simulink model "InstCamberStiffness"  (R2024b)
settings: Solver=VariableStepAuto  StartTime=0.0  StopTime=30  RelTol=1e-3
libraries: simulink x1
settings Model: Creator=owen  LastModifiedBy=owen

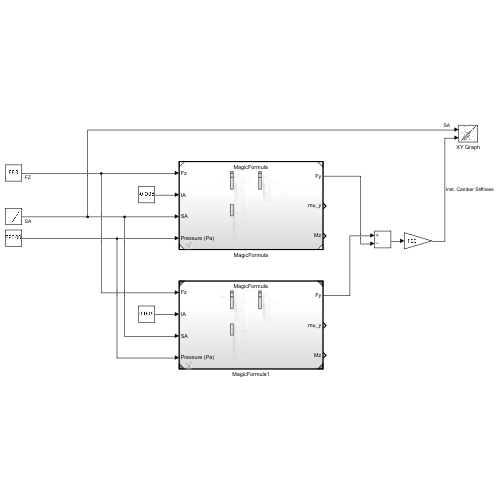
[thumbnail: Simulink's stored preview of the top-level diagram]
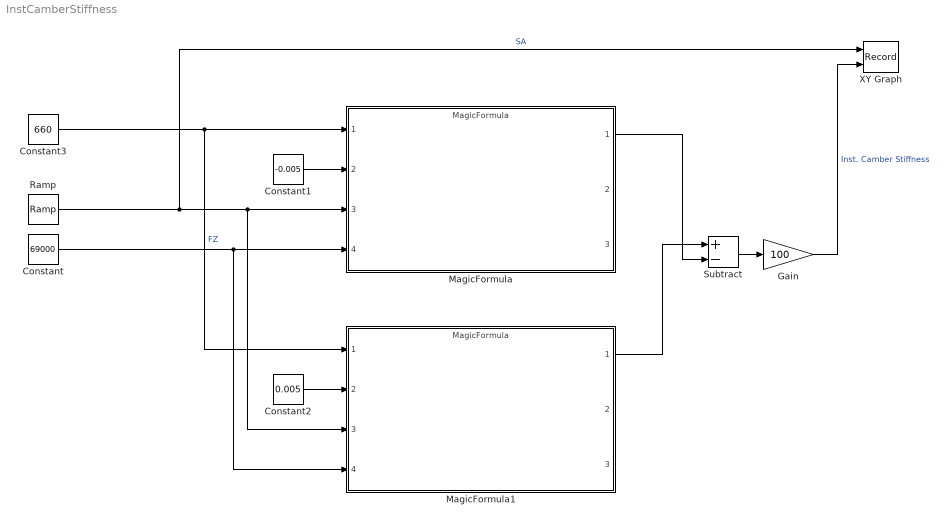
== system InstCamberStiffness ==
  Constant : Constant  Value=69000
  Constant1 : Constant  Value=-0.005
  Constant2 : Constant  Value=0.005
  Constant3 : Constant  Value=660
  Gain : Gain  Gain=100
  MagicFormula : ModelReference  ModelNameDialog=MagicFormula.slx  SimulationMode=Normal  ModelReferenceVersion=1.53
  MagicFormula1 : ModelReference  ModelNameDialog=MagicFormula.slx  SimulationMode=Normal  ModelReferenceVersion=1.53
  Ramp : simulink/Sources/Ramp  slope=1  start=0  InitialOutput=-15
  Subtract : Sum  Inputs=+-
  XY Graph : Record  FileSettingsInternal="{\"entries\":[{\"content\":{\"excelSettings\":{\"content\":{},\"type\":\"Streamout.ExcelSettings\"}},\"type\":\"Streamout.FileSettingStorage\",\"uuid\":\"\"}],\"packageUris\":[\"http:\\/\\/schema.mathworks.com\\/mf0\\/streamout_blocks\\/R2020a\"],\"version\":\"1.0\"}"  Layout=[1 1]  SignalsInternal="{\"entries\":[{\"content\":{\"signals\":[{\"content\":{\"blockPath\":[],\"dimensions\":[1],\"domain\":\"\",\"lineColor\":\"#a2142f\",\"plots\":[ 1 ],\"port\":1,\"sid\":[\"\"],\"signalID\":1,\"signalName\":\"SA\"},\"type\":\"RecordBlkView.Signal\",\"uuid\":\"\"},{\"content\":{\"blockPath\":[],\"dimensions\":[1],\"domain\":\"\",\"lineColor\":\"#139fff\",\"plots\":[ 1 ],\"port\":2,\"sid\":[\"\"],\"signalID\":2,\"signalName\":\"Inst. Camber Stiffness\"},\"type\":\"RecordBlkView.Signal\",\"uuid\":\"\"}]},\"type\":\"RecordBlkView.InputSignals\",\"uuid\":\"\"}],\"packageUris\":[\"http:\\/\\/schema.mathworks.com\\/mf0\\/streamout_blocks\\/R2020a\"],\"version\":\"1.0\"}"  VisualizationBindings="{\"xyplotplugin\":{\"info\":[{\"series\":[{\"bindingParametersList\":[{\"parameter\":\"X-Axis\",\"signalID\":1,\"signalName\":\"SA\"},{\"parameter\":\"Y-Axis\",\"signalID\":2,\"signalName\":\"Inst. Camber Stiffness\"}],\"seriesID\":0}],\"subplotID\":1}]}}"  CompatibilityTag=XY
  wires:
  Constant/1 -> MagicFormula1/4, MagicFormula/4
  Constant1/1 -> MagicFormula/2
  Constant2/1 -> MagicFormula1/2
  Ramp/1 -> XY Graph/1, MagicFormula1/3, MagicFormula/3  "SA"
  Constant3/1 -> MagicFormula1/1, MagicFormula/1  "FZ"
  MagicFormula/1 -> Subtract/2
  MagicFormula1/1 -> Subtract/1
  Subtract/1 -> Gain/1
  Gain/1 -> XY Graph/2  "Inst. Camber Stiffness"
